simulink model "CH23_3D"  (R2021b)
settings: Solver=ode45  StartTime=0.0  StopTime=50  RelTol=1e-3  EnableMultiTasking=on
libraries: simulink x6, commrandsrc2 x2, commdigbbndam3 x2, commfilt2 x2
settings Model: Creator=my2  LastModifiedBy=82102
settings SolverCC: AlgebraicLoopSolver=TrustRegion
settings DataIOCC: LimitDataPoints=on  SaveFormat=Array  SignalLoggingSaveFormat=ModelDataLogs  ReturnWorkspaceOutputs=off
settings OptimizationCC: LifeSpan=inf
settings DebuggingCC: SolverPrmCheckMsg=warning  MultiTaskDSMMsg=warning  MultiTaskCondExecSysMsg=none  FcnCallInpInsideContextMsg=warning  SFUnexpectedBacktrackingDiag=warning  SFNoUnconditionalDefaultTransitionDiag=warning  SFExecutionAtInitializationDiag=none  SFMachineParentedDataDiag=warning  ArithmeticOperatorsInVariantConditions=warning
settings HardwareCC: ProdBitPerPointer=32  ProdBitPerSizeT=32  ProdBitPerPtrDiffT=32  ProdLargestAtomicFloat=None  ProdIntDivRoundTo=Undefined  ProdEndianess=Unspecified  ProdWordSize=32  ProdHWDeviceType=32-bit Generic
settings ModelReferenceCC: PropagateSignalLabelsOutOfModel=off
settings SFSimCC: SimUseLocalCustomCode=off  CustomCodeUndefinedFunction=UseInterfaceOnly
settings RTWCC: RTWUseLocalCustomCode=off
settings CodeAppCC: StateflowObjectComments=on
settings GRTTargetCC: TargetLangStandard=C89/C90 (ANSI)  CombineOutputUpdateFcns=off  GRTInterface=on
settings ConfigComp: CovMetricSettings=dw  CovSaveCumulativeToWorkspaceVar=on  CovSaveSingleToWorkspaceVar=on  CovExternalEMLEnable=off

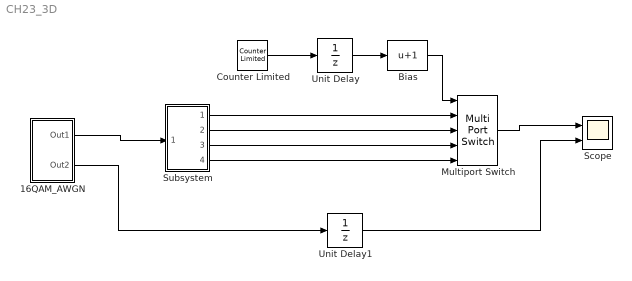
== system CH23_3D ==
  16QAM_AWGN : Subsystem
  Bias : Bias  Bias=1
  Counter Limited : simulink/Sources/Counter Limited  uplimit=3  tsamp=-1
  Multiport Switch : MultiPortSwitch  Inputs=4
  Scope : Scope  NumInputPorts=2
  Subsystem : Subsystem
  Unit Delay : UnitDelay
  Unit Delay1 : UnitDelay
  wires:
  Counter Limited/1 -> Unit Delay/1
  Unit Delay/1 -> Bias/1
  Subsystem/1(Out1) -> Multiport Switch/2
  Subsystem/2(Out2) -> Multiport Switch/3
  Subsystem/3(Out3) -> Multiport Switch/4
  Subsystem/4(Out4) -> Multiport Switch/5
  Bias/1 -> Multiport Switch/1
  16QAM_AWGN/2(Out2) -> Unit Delay1/1
  Unit Delay1/1 -> Scope/2
  Multiport Switch/1 -> Scope/1
  16QAM_AWGN/1(Out1) -> Subsystem/1(In1)

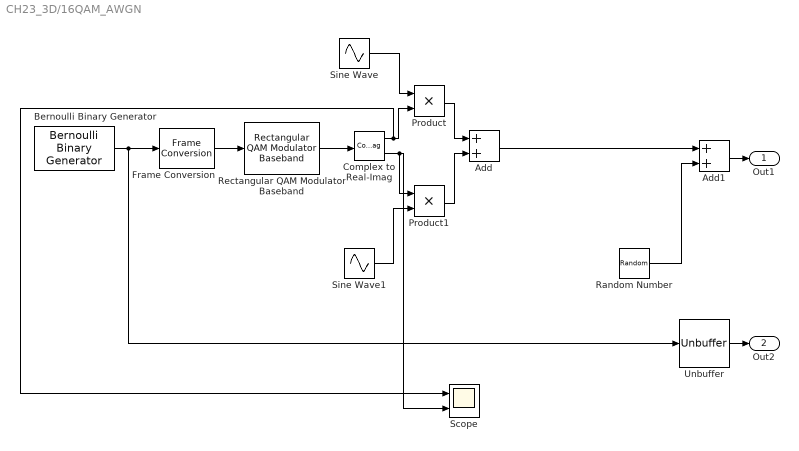
== system CH23_3D/16QAM_AWGN ==
  Add : Sum
  Add1 : Sum
  Bernoulli Binary Generator : commrandsrc2/Bernoulli Binary Generator  P=0.5  seed=20301181  Ts=1  frameBased=on  sampPerFrame=4  orient=off  outDataType=boolean
      settings: SourceProductBaseCode=CM
  Complex to Real-Imag : ComplexToRealImag
  Frame Conversion : FrameConversion  OutFrame=Sample-based
  Product : Product
  Product1 : Product
  Random Number : RandomNumber  Variance=10*0  Seed=41  SampleTime=1/100  VectorParams1D=off
  Rectangular QAM Modulator Baseband : commdigbbndam3/Rectangular QAM Modulator Baseband  M=16  InType=Bit  Enc=Gray  Mapping=[0:15]  PowType=Min. distance between symbols  MinDist=2  AvgPow=1  PeakPow=1  Ph=0  outDtype=double  outWordLen=16  outUDDataType=sfix(16)  outFracLenMode=Best precision  outFracLen=15  outDataTypeStr=double  outLastDataTypeStr=double
  Scope : Scope  NumInputPorts=2
  Sine Wave : Sin  SampleTime=1/100
  Sine Wave1 : Sin  SampleTime=1/100
  Unbuffer : Unbuffer
  Out1 : Outport
  Out2 : Outport  Port=2
  wires:
  Complex to Real-Imag/2 -> Scope/2, Product1/1
  Unbuffer/1 -> Out2/1
  Add1/1 -> Out1/1
  Random Number/1 -> Add1/2
  Complex to Real-Imag/1 -> Scope/1, Product/2
  Sine Wave/1 -> Product/1
  Rectangular QAM Modulator Baseband/1 -> Complex to Real-Imag/1
  Frame Conversion/1 -> Rectangular QAM Modulator Baseband/1
  Bernoulli Binary Generator/1 -> Frame Conversion/1, Unbuffer/1
  Product/1 -> Add/1
  Sine Wave1/1 -> Product1/2
  Add/1 -> Add1/1
  Product1/1 -> Add/2

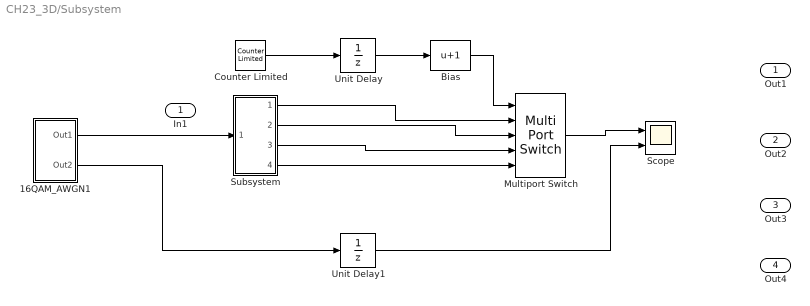
== system CH23_3D/Subsystem ==
  In1 : Inport
  16QAM_AWGN1 : Subsystem
  Bias : Bias  Bias=1
  Counter Limited : simulink/Sources/Counter Limited  uplimit=3  tsamp=-1
  Multiport Switch : MultiPortSwitch  Inputs=4
  Scope : Scope  NumInputPorts=2
  Subsystem : Subsystem
  Unit Delay : UnitDelay  HasFrameUpgradeWarning=on
  Unit Delay1 : UnitDelay  HasFrameUpgradeWarning=on
  Out1 : Outport
  Out2 : Outport  Port=2
  Out3 : Outport  Port=3
  Out4 : Outport  Port=4
  wires:
  16QAM_AWGN1/1(Out1) -> Subsystem/1(In1)
  Counter Limited/1 -> Unit Delay/1
  Unit Delay/1 -> Bias/1
  16QAM_AWGN1/2(Out2) -> Unit Delay1/1
  Subsystem/1(Out1) -> Multiport Switch/2
  Subsystem/2(Out2) -> Multiport Switch/3
  Subsystem/3(Out3) -> Multiport Switch/4
  Subsystem/4(Out4) -> Multiport Switch/5
  Bias/1 -> Multiport Switch/1
  Multiport Switch/1 -> Scope/1
  Unit Delay1/1 -> Scope/2

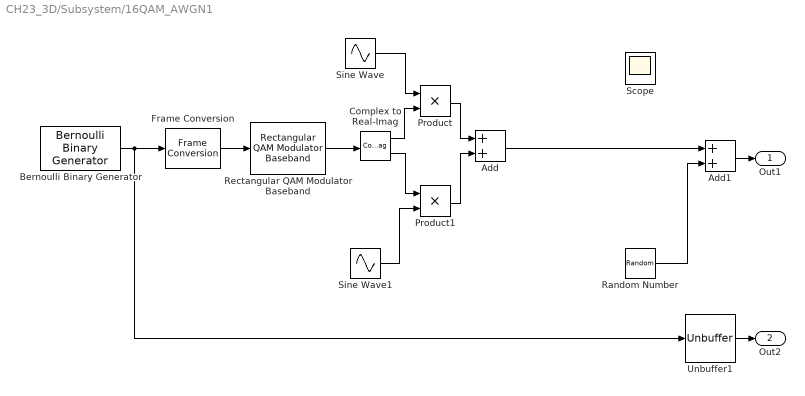
== system CH23_3D/Subsystem/16QAM_AWGN1 ==
  Add : Sum
  Add1 : Sum
  Bernoulli Binary Generator : commrandsrc2/Bernoulli Binary Generator  P=0.5  seed=22012225  Ts=1  frameBased=on  sampPerFrame=4  orient=off  outDataType=boolean
      settings: SourceProductBaseCode=CM
  Complex to Real-Imag : ComplexToRealImag
  Frame Conversion : FrameConversion  OutFrame=Sample-based
  Product : Product
  Product1 : Product
  Random Number : RandomNumber  Variance=0  Seed=41  SampleTime=1/100  VectorParams1D=off
  Rectangular QAM Modulator Baseband : commdigbbndam3/Rectangular QAM Modulator Baseband  M=16  InType=Bit  Enc=Gray  Mapping=[0:15]  PowType=Min. distance between symbols  MinDist=2  AvgPow=1  PeakPow=1  Ph=0  outDtype=double  outWordLen=16  outUDDataType=sfix(16)  outFracLenMode=Best precision  outFracLen=15  outDataTypeStr=double  outLastDataTypeStr=double
  Scope : Scope
  Sine Wave : Sin  Amplitude=sqrt(2)  Frequency=2*pi*20  Phase=pi/2  SampleTime=1/100
  Sine Wave1 : Sin  Amplitude=sqrt(2)  Frequency=2*pi*20  SampleTime=1/100
  Unbuffer1 : Unbuffer
  Out1 : Outport
  Out2 : Outport  Port=2
  wires:
  Bernoulli Binary Generator/1 -> Frame Conversion/1, Unbuffer1/1
  Complex to Real-Imag/2 -> Product1/1
  Unbuffer1/1 -> Out2/1
  Product1/1 -> Add/2
  Random Number/1 -> Add1/2
  Add/1 -> Add1/1
  Product/1 -> Add/1
  Rectangular QAM Modulator Baseband/1 -> Complex to Real-Imag/1
  Complex to Real-Imag/1 -> Product/2
  Sine Wave1/1 -> Product1/2
  Frame Conversion/1 -> Rectangular QAM Modulator Baseband/1
  Sine Wave/1 -> Product/1
  Add1/1 -> Out1/1

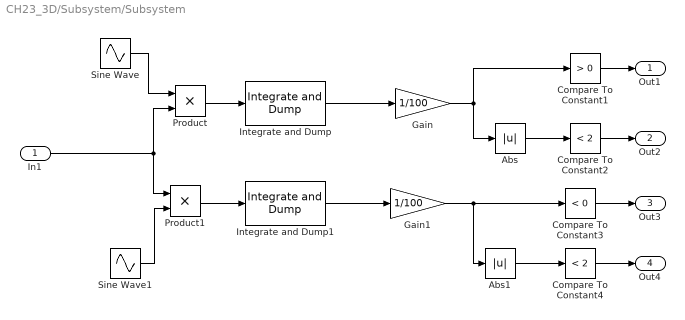
== system CH23_3D/Subsystem/Subsystem ==
  In1 : Inport
  Abs : Abs
  Abs1 : Abs
  Compare To Constant1 : simulink/Logic and Bit Operations/Compare To Constant  relop=>  const=0  OutDataTypeStr=boolean
  Compare To Constant2 : simulink/Logic and Bit Operations/Compare To Constant  relop=<  const=2  OutDataTypeStr=boolean
  Compare To Constant3 : simulink/Logic and Bit Operations/Compare To Constant  relop=<  const=0  OutDataTypeStr=boolean
  Compare To Constant4 : simulink/Logic and Bit Operations/Compare To Constant  relop=<  const=2  OutDataTypeStr=boolean
  Gain : Gain  Gain=1/100
  Gain1 : Gain  Gain=1/100
  Integrate and Dump : commfilt2/Integrate and Dump  obssamples=100  offsetsamples=0  nodump=off  roundingMode=Floor  overflowMode=off  outputDataTypeStr=Inherit: Same as accumulator  outputLastDataTypeStr=Inherit: Same as accumulator
  Integrate and Dump1 : commfilt2/Integrate and Dump  obssamples=100  offsetsamples=0  nodump=off  roundingMode=Floor  overflowMode=off  outputDataTypeStr=Inherit: Same as accumulator  outputLastDataTypeStr=Inherit: Same as accumulator
  Product : Product
  Product1 : Product
  Sine Wave : Sin  Amplitude=sqrt(2)  Frequency=2*pi*20  Phase=pi/2  SampleTime=1/100
  Sine Wave1 : Sin  Amplitude=sqrt(2)  Frequency=2*pi*20  SampleTime=1/100
  Out1 : Outport
  Out2 : Outport  Port=2
  Out3 : Outport  Port=3
  Out4 : Outport  Port=4
  wires:
  Product/1 -> Integrate and Dump/1
  Gain/1 -> Abs/1, Compare To Constant1/1
  Gain1/1 -> Abs1/1, Compare To Constant3/1
  Integrate and Dump/1 -> Gain/1
  Compare To Constant3/1 -> Out3/1
  Compare To Constant4/1 -> Out4/1
  Compare To Constant2/1 -> Out2/1
  In1/1 -> Product1/1, Product/2
  Sine Wave/1 -> Product/1
  Product1/1 -> Integrate and Dump1/1
  Compare To Constant1/1 -> Out1/1
  Sine Wave1/1 -> Product1/2
  Abs/1 -> Compare To Constant2/1
  Abs1/1 -> Compare To Constant4/1
  Integrate and Dump1/1 -> Gain1/1
